simulink model "lab4"  (R2016b)
settings: Solver=VariableStepAuto  StartTime=0.0  StopTime=totaltime  RelTol=1e-3
undefined symbols (not defined in the file or in its folder): h, st
libraries: xbsIndex_r4 x1191
(part 2 of 3)

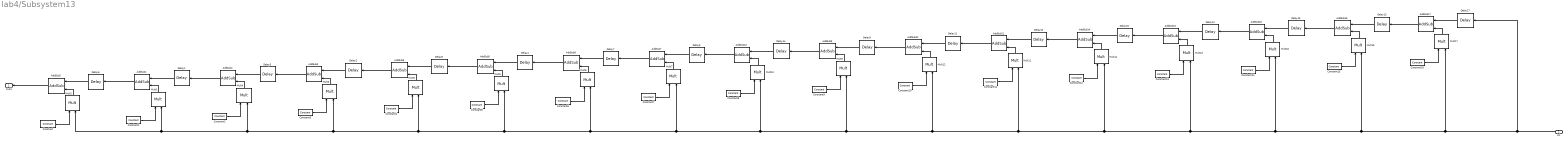
== system lab4/Subsystem13 ==
  In1 : Inport
  AddSub{1..17} (17 alike) : xbsIndex_r4/AddSub  mode=Addition  use_carryin=off  use_carryout=off  en=off  latency=0  precision=User Defined  arith_type="Signed  (2's comp)"  n_bits=17  bin_pt=14  quantization=Truncate  overflow=Wrap  use_behavioral_HDL=off  hw_selection=Fabric  pipelined=off  dbl_ovrd=off  block_type=addsub
  Constant : xbsIndex_r4/Constant  const=h(4,17)  gui_display_data_type=Fixed-point  arith_type=Signed (2's comp)  n_bits=16  bin_pt=14  preci_type=Single  exp_width=8  frac_width=24  explicit_period=off  period=1  equ=P=C  opselect=C  inp2=PCIN>>17  opr=+  inp1=P  carry=CIN  dbl_ovrd=off  block_type=constant
  Constant1 : xbsIndex_r4/Constant  const=h(4,16)  gui_display_data_type=Fixed-point  arith_type=Signed (2's comp)  n_bits=16  bin_pt=14  preci_type=Single  exp_width=8  frac_width=24  explicit_period=off  period=1  equ=P=C  opselect=C  inp2=PCIN>>17  opr=+  inp1=P  carry=CIN  dbl_ovrd=off  block_type=constant
  Constant10 : xbsIndex_r4/Constant  const=h(4,7)  gui_display_data_type=Fixed-point  arith_type=Signed (2's comp)  n_bits=16  bin_pt=14  preci_type=Single  exp_width=8  frac_width=24  explicit_period=off  period=1  equ=P=C  opselect=C  inp2=PCIN>>17  opr=+  inp1=P  carry=CIN  dbl_ovrd=off  block_type=constant
  Constant11 : xbsIndex_r4/Constant  const=h(4,6)  gui_display_data_type=Fixed-point  arith_type=Signed (2's comp)  n_bits=16  bin_pt=14  preci_type=Single  exp_width=8  frac_width=24  explicit_period=off  period=1  equ=P=C  opselect=C  inp2=PCIN>>17  opr=+  inp1=P  carry=CIN  dbl_ovrd=off  block_type=constant
  Constant12 : xbsIndex_r4/Constant  const=h(4,5)  gui_display_data_type=Fixed-point  arith_type=Signed (2's comp)  n_bits=16  bin_pt=14  preci_type=Single  exp_width=8  frac_width=24  explicit_period=off  period=1  equ=P=C  opselect=C  inp2=PCIN>>17  opr=+  inp1=P  carry=CIN  dbl_ovrd=off  block_type=constant
  Constant13 : xbsIndex_r4/Constant  const=h(4,4)  gui_display_data_type=Fixed-point  arith_type=Signed (2's comp)  n_bits=16  bin_pt=14  preci_type=Single  exp_width=8  frac_width=24  explicit_period=off  period=1  equ=P=C  opselect=C  inp2=PCIN>>17  opr=+  inp1=P  carry=CIN  dbl_ovrd=off  block_type=constant
  Constant14 : xbsIndex_r4/Constant  const=h(4,3)  gui_display_data_type=Fixed-point  arith_type=Signed (2's comp)  n_bits=16  bin_pt=14  preci_type=Single  exp_width=8  frac_width=24  explicit_period=off  period=1  equ=P=C  opselect=C  inp2=PCIN>>17  opr=+  inp1=P  carry=CIN  dbl_ovrd=off  block_type=constant
  Constant15 : xbsIndex_r4/Constant  const=h(4,2)  gui_display_data_type=Fixed-point  arith_type=Signed (2's comp)  n_bits=16  bin_pt=14  preci_type=Single  exp_width=8  frac_width=24  explicit_period=off  period=1  equ=P=C  opselect=C  inp2=PCIN>>17  opr=+  inp1=P  carry=CIN  dbl_ovrd=off  block_type=constant
  Constant16 : xbsIndex_r4/Constant  const=h(4,1)  gui_display_data_type=Fixed-point  arith_type=Signed (2's comp)  n_bits=17  bin_pt=14  preci_type=Single  exp_width=8  frac_width=24  explicit_period=off  period=1  equ=P=C  opselect=C  inp2=PCIN>>17  opr=+  inp1=P  carry=CIN  dbl_ovrd=off  block_type=constant
  Constant2 : xbsIndex_r4/Constant  const=h(4,15)  gui_display_data_type=Fixed-point  arith_type=Signed (2's comp)  n_bits=16  bin_pt=14  preci_type=Single  exp_width=8  frac_width=24  explicit_period=off  period=1  equ=P=C  opselect=C  inp2=PCIN>>17  opr=+  inp1=P  carry=CIN  dbl_ovrd=off  block_type=constant
  Constant3 : xbsIndex_r4/Constant  const=h(4,14)  gui_display_data_type=Fixed-point  arith_type=Signed (2's comp)  n_bits=16  bin_pt=14  preci_type=Single  exp_width=8  frac_width=24  explicit_period=off  period=1  equ=P=C  opselect=C  inp2=PCIN>>17  opr=+  inp1=P  carry=CIN  dbl_ovrd=off  block_type=constant
  Constant4 : xbsIndex_r4/Constant  const=h(4,13)  gui_display_data_type=Fixed-point  arith_type=Signed (2's comp)  n_bits=16  bin_pt=14  preci_type=Single  exp_width=8  frac_width=24  explicit_period=off  period=1  equ=P=C  opselect=C  inp2=PCIN>>17  opr=+  inp1=P  carry=CIN  dbl_ovrd=off  block_type=constant
  Constant5 : xbsIndex_r4/Constant  const=h(4,12)  gui_display_data_type=Fixed-point  arith_type=Signed (2's comp)  n_bits=16  bin_pt=14  preci_type=Single  exp_width=8  frac_width=24  explicit_period=off  period=1  equ=P=C  opselect=C  inp2=PCIN>>17  opr=+  inp1=P  carry=CIN  dbl_ovrd=off  block_type=constant
  Constant6 : xbsIndex_r4/Constant  const=h(4,11)  gui_display_data_type=Fixed-point  arith_type=Signed (2's comp)  n_bits=16  bin_pt=14  preci_type=Single  exp_width=8  frac_width=24  explicit_period=off  period=1  equ=P=C  opselect=C  inp2=PCIN>>17  opr=+  inp1=P  carry=CIN  dbl_ovrd=off  block_type=constant
  Constant7 : xbsIndex_r4/Constant  const=h(4,10)  gui_display_data_type=Fixed-point  arith_type=Signed (2's comp)  n_bits=16  bin_pt=14  preci_type=Single  exp_width=8  frac_width=24  explicit_period=off  period=1  equ=P=C  opselect=C  inp2=PCIN>>17  opr=+  inp1=P  carry=CIN  dbl_ovrd=off  block_type=constant
  Constant8 : xbsIndex_r4/Constant  const=h(4,9)  gui_display_data_type=Fixed-point  arith_type=Signed (2's comp)  n_bits=16  bin_pt=14  preci_type=Single  exp_width=8  frac_width=24  explicit_period=off  period=1  equ=P=C  opselect=C  inp2=PCIN>>17  opr=+  inp1=P  carry=CIN  dbl_ovrd=off  block_type=constant
  Constant9 : xbsIndex_r4/Constant  const=h(4,8)  gui_display_data_type=Fixed-point  arith_type=Signed (2's comp)  n_bits=16  bin_pt=14  preci_type=Single  exp_width=8  frac_width=24  explicit_period=off  period=1  equ=P=C  opselect=C  inp2=PCIN>>17  opr=+  inp1=P  carry=CIN  dbl_ovrd=off  block_type=constant
  Delay{1..17} (17 alike) : xbsIndex_r4/Delay  rst=off  infoeditControl=Selection of Reset will increase slice count due to use of real FFs and instead of SRLs  en=off  latency=1  reg_retiming=off  dbl_ovrd=off  block_type=delay
  Mult{1..17} (17 alike) : xbsIndex_r4/Mult  precision=User Defined  arith_type="Signed  (2's comp)"  n_bits=16  bin_pt=14  quantization="Round  (unbiased: +/- Inf)"  overflow=Flag as error  en=off  latency=0  use_behavioral_HDL=off  opt=Speed  use_embedded=on  optimum_pipeline=off  pipeline=on  dbl_ovrd=off  use_rpm=on  placement_style=Triangular  block_type=mult
  Out1 : Outport
  wires:
  Mult2/1 -> AddSub2/2
  AddSub2/1 -> Out1/1
  Delay6/1 -> AddSub2/1
  Constant2/1 -> Mult4/1
  AddSub4/1 -> Delay1/1
  Mult4/1 -> AddSub4/2
  Delay3/1 -> AddSub4/1
  Constant4/1 -> Mult6/1
  AddSub12/1 -> Delay9/1
  Constant3/1 -> Mult3/1
  Mult13/1 -> AddSub13/2
  AddSub13/1 -> Delay16/1
  Delay7/1 -> AddSub8/1
  Constant13/1 -> Mult13/1
  Mult3/1 -> AddSub3/2
  Mult8/1 -> AddSub8/2
  Delay8/1 -> AddSub6/1
  Delay2/1 -> AddSub3/1
  AddSub3/1 -> Delay3/1
  Delay14/1 -> AddSub10/1
  AddSub11/1 -> Delay11/1
  AddSub9/1 -> Delay14/1
  AddSub6/1 -> Delay2/1
  Delay5/1 -> AddSub7/1
  Constant7/1 -> Mult7/1
  Mult5/1 -> AddSub5/2
  Constant5/1 -> Mult5/1
  Mult12/1 -> AddSub12/2
  Mult7/1 -> AddSub7/2
  AddSub7/1 -> Delay7/1
  Delay11/1 -> AddSub12/1
  Mult11/1 -> AddSub11/2
  AddSub8/1 -> Delay4/1
  Delay4/1 -> AddSub5/1
  Constant6/1 -> Mult8/1
  Mult6/1 -> AddSub6/2
  AddSub5/1 -> Delay8/1
  Delay15/1 -> AddSub16/1
  AddSub10/1 -> Delay5/1
  Delay9/1 -> AddSub9/1
  Mult10/1 -> AddSub10/2
  Delay16/1 -> AddSub14/1
  Delay13/1 -> AddSub15/1
  Mult9/1 -> AddSub9/2
  Constant8/1 -> Mult10/1
  Constant15/1 -> Mult15/1
  Constant12/1 -> Mult14/1
  Delay10/1 -> AddSub11/1
  Delay12/1 -> AddSub13/1
  AddSub16/1 -> Delay12/1
  Mult15/1 -> AddSub15/2
  AddSub14/1 -> Delay10/1
  Mult16/1 -> AddSub16/2
  Mult14/1 -> AddSub14/2
  Constant11/1 -> Mult11/1
  Constant9/1 -> Mult9/1
  AddSub15/1 -> Delay15/1
  Constant10/1 -> Mult12/1
  Constant14/1 -> Mult16/1
  In1/1 -> Delay17/1, Mult17/2, Mult15/2, Mult16/2, Mult13/2, Mult14/2, Mult11/2, Mult12/2, Mult9/2, Mult10/2, Mult7/2, Mult8/2, Mult5/2, Mult6/2, Mult3/2, Mult4/2, Mult2/2, Mult1/2
  Delay17/1 -> AddSub17/1
  AddSub17/1 -> Delay13/1
  Mult17/1 -> AddSub17/2
  Constant16/1 -> Mult17/1
  Constant/1 -> Mult2/1
  Delay1/1 -> AddSub1/1
  Mult1/1 -> AddSub1/2
  Constant1/1 -> Mult1/1
  AddSub1/1 -> Delay6/1

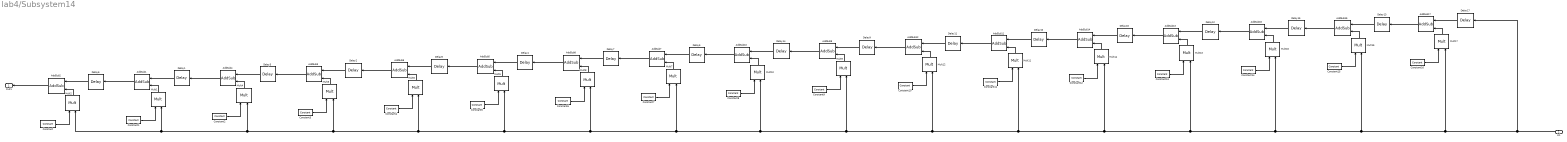
== system lab4/Subsystem14 ==
  In1 : Inport
  AddSub{1..17} (17 alike) : xbsIndex_r4/AddSub  mode=Addition  use_carryin=off  use_carryout=off  en=off  latency=0  precision=User Defined  arith_type="Signed  (2's comp)"  n_bits=17  bin_pt=14  quantization=Truncate  overflow=Wrap  use_behavioral_HDL=off  hw_selection=Fabric  pipelined=off  dbl_ovrd=off  block_type=addsub
  Constant : xbsIndex_r4/Constant  const=h(3,17)  gui_display_data_type=Fixed-point  arith_type=Signed (2's comp)  n_bits=16  bin_pt=14  preci_type=Single  exp_width=8  frac_width=24  explicit_period=off  period=1  equ=P=C  opselect=C  inp2=PCIN>>17  opr=+  inp1=P  carry=CIN  dbl_ovrd=off  block_type=constant
  Constant1 : xbsIndex_r4/Constant  const=h(3,16)  gui_display_data_type=Fixed-point  arith_type=Signed (2's comp)  n_bits=16  bin_pt=14  preci_type=Single  exp_width=8  frac_width=24  explicit_period=off  period=1  equ=P=C  opselect=C  inp2=PCIN>>17  opr=+  inp1=P  carry=CIN  dbl_ovrd=off  block_type=constant
  Constant10 : xbsIndex_r4/Constant  const=h(3,7)  gui_display_data_type=Fixed-point  arith_type=Signed (2's comp)  n_bits=16  bin_pt=14  preci_type=Single  exp_width=8  frac_width=24  explicit_period=off  period=1  equ=P=C  opselect=C  inp2=PCIN>>17  opr=+  inp1=P  carry=CIN  dbl_ovrd=off  block_type=constant
  Constant11 : xbsIndex_r4/Constant  const=h(3,6)  gui_display_data_type=Fixed-point  arith_type=Signed (2's comp)  n_bits=16  bin_pt=14  preci_type=Single  exp_width=8  frac_width=24  explicit_period=off  period=1  equ=P=C  opselect=C  inp2=PCIN>>17  opr=+  inp1=P  carry=CIN  dbl_ovrd=off  block_type=constant
  Constant12 : xbsIndex_r4/Constant  const=h(3,5)  gui_display_data_type=Fixed-point  arith_type=Signed (2's comp)  n_bits=16  bin_pt=14  preci_type=Single  exp_width=8  frac_width=24  explicit_period=off  period=1  equ=P=C  opselect=C  inp2=PCIN>>17  opr=+  inp1=P  carry=CIN  dbl_ovrd=off  block_type=constant
  Constant13 : xbsIndex_r4/Constant  const=h(3,4)  gui_display_data_type=Fixed-point  arith_type=Signed (2's comp)  n_bits=16  bin_pt=14  preci_type=Single  exp_width=8  frac_width=24  explicit_period=off  period=1  equ=P=C  opselect=C  inp2=PCIN>>17  opr=+  inp1=P  carry=CIN  dbl_ovrd=off  block_type=constant
  Constant14 : xbsIndex_r4/Constant  const=h(3,3)  gui_display_data_type=Fixed-point  arith_type=Signed (2's comp)  n_bits=16  bin_pt=14  preci_type=Single  exp_width=8  frac_width=24  explicit_period=off  period=1  equ=P=C  opselect=C  inp2=PCIN>>17  opr=+  inp1=P  carry=CIN  dbl_ovrd=off  block_type=constant
  Constant15 : xbsIndex_r4/Constant  const=h(3,2)  gui_display_data_type=Fixed-point  arith_type=Signed (2's comp)  n_bits=16  bin_pt=14  preci_type=Single  exp_width=8  frac_width=24  explicit_period=off  period=1  equ=P=C  opselect=C  inp2=PCIN>>17  opr=+  inp1=P  carry=CIN  dbl_ovrd=off  block_type=constant
  Constant16 : xbsIndex_r4/Constant  const=h(3,1)  gui_display_data_type=Fixed-point  arith_type=Signed (2's comp)  n_bits=17  bin_pt=14  preci_type=Single  exp_width=8  frac_width=24  explicit_period=off  period=1  equ=P=C  opselect=C  inp2=PCIN>>17  opr=+  inp1=P  carry=CIN  dbl_ovrd=off  block_type=constant
  Constant2 : xbsIndex_r4/Constant  const=h(3,15)  gui_display_data_type=Fixed-point  arith_type=Signed (2's comp)  n_bits=16  bin_pt=14  preci_type=Single  exp_width=8  frac_width=24  explicit_period=off  period=1  equ=P=C  opselect=C  inp2=PCIN>>17  opr=+  inp1=P  carry=CIN  dbl_ovrd=off  block_type=constant
  Constant3 : xbsIndex_r4/Constant  const=h(3,14)  gui_display_data_type=Fixed-point  arith_type=Signed (2's comp)  n_bits=16  bin_pt=14  preci_type=Single  exp_width=8  frac_width=24  explicit_period=off  period=1  equ=P=C  opselect=C  inp2=PCIN>>17  opr=+  inp1=P  carry=CIN  dbl_ovrd=off  block_type=constant
  Constant4 : xbsIndex_r4/Constant  const=h(3,13)  gui_display_data_type=Fixed-point  arith_type=Signed (2's comp)  n_bits=16  bin_pt=14  preci_type=Single  exp_width=8  frac_width=24  explicit_period=off  period=1  equ=P=C  opselect=C  inp2=PCIN>>17  opr=+  inp1=P  carry=CIN  dbl_ovrd=off  block_type=constant
  Constant5 : xbsIndex_r4/Constant  const=h(3,12)  gui_display_data_type=Fixed-point  arith_type=Signed (2's comp)  n_bits=16  bin_pt=14  preci_type=Single  exp_width=8  frac_width=24  explicit_period=off  period=1  equ=P=C  opselect=C  inp2=PCIN>>17  opr=+  inp1=P  carry=CIN  dbl_ovrd=off  block_type=constant
  Constant6 : xbsIndex_r4/Constant  const=h(3,11)  gui_display_data_type=Fixed-point  arith_type=Signed (2's comp)  n_bits=16  bin_pt=14  preci_type=Single  exp_width=8  frac_width=24  explicit_period=off  period=1  equ=P=C  opselect=C  inp2=PCIN>>17  opr=+  inp1=P  carry=CIN  dbl_ovrd=off  block_type=constant
  Constant7 : xbsIndex_r4/Constant  const=h(3,10)  gui_display_data_type=Fixed-point  arith_type=Signed (2's comp)  n_bits=16  bin_pt=14  preci_type=Single  exp_width=8  frac_width=24  explicit_period=off  period=1  equ=P=C  opselect=C  inp2=PCIN>>17  opr=+  inp1=P  carry=CIN  dbl_ovrd=off  block_type=constant
  Constant8 : xbsIndex_r4/Constant  const=h(3,9)  gui_display_data_type=Fixed-point  arith_type=Signed (2's comp)  n_bits=16  bin_pt=14  preci_type=Single  exp_width=8  frac_width=24  explicit_period=off  period=1  equ=P=C  opselect=C  inp2=PCIN>>17  opr=+  inp1=P  carry=CIN  dbl_ovrd=off  block_type=constant
  Constant9 : xbsIndex_r4/Constant  const=h(3,8)  gui_display_data_type=Fixed-point  arith_type=Signed (2's comp)  n_bits=16  bin_pt=14  preci_type=Single  exp_width=8  frac_width=24  explicit_period=off  period=1  equ=P=C  opselect=C  inp2=PCIN>>17  opr=+  inp1=P  carry=CIN  dbl_ovrd=off  block_type=constant
  Delay{1..17} (17 alike) : xbsIndex_r4/Delay  rst=off  infoeditControl=Selection of Reset will increase slice count due to use of real FFs and instead of SRLs  en=off  latency=1  reg_retiming=off  dbl_ovrd=off  block_type=delay
  Mult{1..17} (17 alike) : xbsIndex_r4/Mult  precision=User Defined  arith_type="Signed  (2's comp)"  n_bits=16  bin_pt=14  quantization="Round  (unbiased: +/- Inf)"  overflow=Flag as error  en=off  latency=0  use_behavioral_HDL=off  opt=Speed  use_embedded=on  optimum_pipeline=off  pipeline=on  dbl_ovrd=off  use_rpm=on  placement_style=Triangular  block_type=mult
  Out1 : Outport
  wires:
  Mult2/1 -> AddSub2/2
  AddSub2/1 -> Out1/1
  Delay6/1 -> AddSub2/1
  Constant2/1 -> Mult4/1
  AddSub4/1 -> Delay1/1
  Mult4/1 -> AddSub4/2
  Delay3/1 -> AddSub4/1
  Constant4/1 -> Mult6/1
  AddSub12/1 -> Delay9/1
  Constant3/1 -> Mult3/1
  Mult13/1 -> AddSub13/2
  AddSub13/1 -> Delay16/1
  Delay7/1 -> AddSub8/1
  Constant13/1 -> Mult13/1
  Mult3/1 -> AddSub3/2
  Mult8/1 -> AddSub8/2
  Delay8/1 -> AddSub6/1
  Delay2/1 -> AddSub3/1
  AddSub3/1 -> Delay3/1
  Delay14/1 -> AddSub10/1
  AddSub11/1 -> Delay11/1
  AddSub9/1 -> Delay14/1
  AddSub6/1 -> Delay2/1
  Delay5/1 -> AddSub7/1
  Constant7/1 -> Mult7/1
  Mult5/1 -> AddSub5/2
  Constant5/1 -> Mult5/1
  Mult12/1 -> AddSub12/2
  Mult7/1 -> AddSub7/2
  AddSub7/1 -> Delay7/1
  Delay11/1 -> AddSub12/1
  Mult11/1 -> AddSub11/2
  AddSub8/1 -> Delay4/1
  Delay4/1 -> AddSub5/1
  Constant6/1 -> Mult8/1
  Mult6/1 -> AddSub6/2
  AddSub5/1 -> Delay8/1
  Delay15/1 -> AddSub16/1
  AddSub10/1 -> Delay5/1
  Delay9/1 -> AddSub9/1
  Mult10/1 -> AddSub10/2
  Delay16/1 -> AddSub14/1
  Delay13/1 -> AddSub15/1
  Mult9/1 -> AddSub9/2
  Constant8/1 -> Mult10/1
  Constant15/1 -> Mult15/1
  Constant12/1 -> Mult14/1
  Delay10/1 -> AddSub11/1
  Delay12/1 -> AddSub13/1
  AddSub16/1 -> Delay12/1
  Mult15/1 -> AddSub15/2
  AddSub14/1 -> Delay10/1
  Mult16/1 -> AddSub16/2
  Mult14/1 -> AddSub14/2
  Constant11/1 -> Mult11/1
  Constant9/1 -> Mult9/1
  AddSub15/1 -> Delay15/1
  Constant10/1 -> Mult12/1
  Constant14/1 -> Mult16/1
  In1/1 -> Delay17/1, Mult17/2, Mult15/2, Mult16/2, Mult13/2, Mult14/2, Mult11/2, Mult12/2, Mult9/2, Mult10/2, Mult7/2, Mult8/2, Mult5/2, Mult6/2, Mult3/2, Mult4/2, Mult2/2, Mult1/2
  Delay17/1 -> AddSub17/1
  AddSub17/1 -> Delay13/1
  Mult17/1 -> AddSub17/2
  Constant16/1 -> Mult17/1
  Constant/1 -> Mult2/1
  Delay1/1 -> AddSub1/1
  Mult1/1 -> AddSub1/2
  Constant1/1 -> Mult1/1
  AddSub1/1 -> Delay6/1

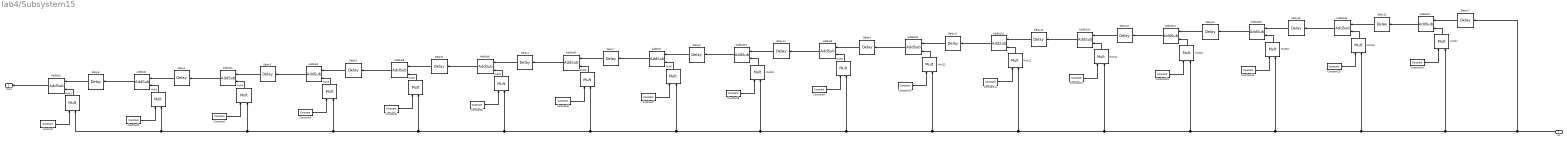
== system lab4/Subsystem15 ==
  In1 : Inport
  AddSub{1..17} (17 alike) : xbsIndex_r4/AddSub  mode=Addition  use_carryin=off  use_carryout=off  en=off  latency=0  precision=User Defined  arith_type="Signed  (2's comp)"  n_bits=17  bin_pt=14  quantization=Truncate  overflow=Wrap  use_behavioral_HDL=off  hw_selection=Fabric  pipelined=off  dbl_ovrd=off  block_type=addsub
  Constant : xbsIndex_r4/Constant  const=h(2,17)  gui_display_data_type=Fixed-point  arith_type=Signed (2's comp)  n_bits=16  bin_pt=14  preci_type=Single  exp_width=8  frac_width=24  explicit_period=off  period=1  equ=P=C  opselect=C  inp2=PCIN>>17  opr=+  inp1=P  carry=CIN  dbl_ovrd=off  block_type=constant
  Constant1 : xbsIndex_r4/Constant  const=h(2,16)  gui_display_data_type=Fixed-point  arith_type=Signed (2's comp)  n_bits=16  bin_pt=14  preci_type=Single  exp_width=8  frac_width=24  explicit_period=off  period=1  equ=P=C  opselect=C  inp2=PCIN>>17  opr=+  inp1=P  carry=CIN  dbl_ovrd=off  block_type=constant
  Constant10 : xbsIndex_r4/Constant  const=h(2,7)  gui_display_data_type=Fixed-point  arith_type=Signed (2's comp)  n_bits=16  bin_pt=14  preci_type=Single  exp_width=8  frac_width=24  explicit_period=off  period=1  equ=P=C  opselect=C  inp2=PCIN>>17  opr=+  inp1=P  carry=CIN  dbl_ovrd=off  block_type=constant
  Constant11 : xbsIndex_r4/Constant  const=h(2,6)  gui_display_data_type=Fixed-point  arith_type=Signed (2's comp)  n_bits=16  bin_pt=14  preci_type=Single  exp_width=8  frac_width=24  explicit_period=off  period=1  equ=P=C  opselect=C  inp2=PCIN>>17  opr=+  inp1=P  carry=CIN  dbl_ovrd=off  block_type=constant
  Constant12 : xbsIndex_r4/Constant  const=h(2,5)  gui_display_data_type=Fixed-point  arith_type=Signed (2's comp)  n_bits=16  bin_pt=14  preci_type=Single  exp_width=8  frac_width=24  explicit_period=off  period=1  equ=P=C  opselect=C  inp2=PCIN>>17  opr=+  inp1=P  carry=CIN  dbl_ovrd=off  block_type=constant
  Constant13 : xbsIndex_r4/Constant  const=h(2,4)  gui_display_data_type=Fixed-point  arith_type=Signed (2's comp)  n_bits=16  bin_pt=14  preci_type=Single  exp_width=8  frac_width=24  explicit_period=off  period=1  equ=P=C  opselect=C  inp2=PCIN>>17  opr=+  inp1=P  carry=CIN  dbl_ovrd=off  block_type=constant
  Constant14 : xbsIndex_r4/Constant  const=h(2,3)  gui_display_data_type=Fixed-point  arith_type=Signed (2's comp)  n_bits=16  bin_pt=14  preci_type=Single  exp_width=8  frac_width=24  explicit_period=off  period=1  equ=P=C  opselect=C  inp2=PCIN>>17  opr=+  inp1=P  carry=CIN  dbl_ovrd=off  block_type=constant
  Constant15 : xbsIndex_r4/Constant  const=h(2,2)  gui_display_data_type=Fixed-point  arith_type=Signed (2's comp)  n_bits=16  bin_pt=14  preci_type=Single  exp_width=8  frac_width=24  explicit_period=off  period=1  equ=P=C  opselect=C  inp2=PCIN>>17  opr=+  inp1=P  carry=CIN  dbl_ovrd=off  block_type=constant
  Constant16 : xbsIndex_r4/Constant  const=h(2,1)  gui_display_data_type=Fixed-point  arith_type=Signed (2's comp)  n_bits=17  bin_pt=14  preci_type=Single  exp_width=8  frac_width=24  explicit_period=off  period=1  equ=P=C  opselect=C  inp2=PCIN>>17  opr=+  inp1=P  carry=CIN  dbl_ovrd=off  block_type=constant
  Constant2 : xbsIndex_r4/Constant  const=h(2,15)  gui_display_data_type=Fixed-point  arith_type=Signed (2's comp)  n_bits=16  bin_pt=14  preci_type=Single  exp_width=8  frac_width=24  explicit_period=off  period=1  equ=P=C  opselect=C  inp2=PCIN>>17  opr=+  inp1=P  carry=CIN  dbl_ovrd=off  block_type=constant
  Constant3 : xbsIndex_r4/Constant  const=h(2,14)  gui_display_data_type=Fixed-point  arith_type=Signed (2's comp)  n_bits=16  bin_pt=14  preci_type=Single  exp_width=8  frac_width=24  explicit_period=off  period=1  equ=P=C  opselect=C  inp2=PCIN>>17  opr=+  inp1=P  carry=CIN  dbl_ovrd=off  block_type=constant
  Constant4 : xbsIndex_r4/Constant  const=h(2,13)  gui_display_data_type=Fixed-point  arith_type=Signed (2's comp)  n_bits=16  bin_pt=14  preci_type=Single  exp_width=8  frac_width=24  explicit_period=off  period=1  equ=P=C  opselect=C  inp2=PCIN>>17  opr=+  inp1=P  carry=CIN  dbl_ovrd=off  block_type=constant
  Constant5 : xbsIndex_r4/Constant  const=h(2,12)  gui_display_data_type=Fixed-point  arith_type=Signed (2's comp)  n_bits=16  bin_pt=14  preci_type=Single  exp_width=8  frac_width=24  explicit_period=off  period=1  equ=P=C  opselect=C  inp2=PCIN>>17  opr=+  inp1=P  carry=CIN  dbl_ovrd=off  block_type=constant
  Constant6 : xbsIndex_r4/Constant  const=h(2,11)  gui_display_data_type=Fixed-point  arith_type=Signed (2's comp)  n_bits=16  bin_pt=14  preci_type=Single  exp_width=8  frac_width=24  explicit_period=off  period=1  equ=P=C  opselect=C  inp2=PCIN>>17  opr=+  inp1=P  carry=CIN  dbl_ovrd=off  block_type=constant
  Constant7 : xbsIndex_r4/Constant  const=h(2,10)  gui_display_data_type=Fixed-point  arith_type=Signed (2's comp)  n_bits=16  bin_pt=14  preci_type=Single  exp_width=8  frac_width=24  explicit_period=off  period=1  equ=P=C  opselect=C  inp2=PCIN>>17  opr=+  inp1=P  carry=CIN  dbl_ovrd=off  block_type=constant
  Constant8 : xbsIndex_r4/Constant  const=h(2,9)  gui_display_data_type=Fixed-point  arith_type=Signed (2's comp)  n_bits=16  bin_pt=14  preci_type=Single  exp_width=8  frac_width=24  explicit_period=off  period=1  equ=P=C  opselect=C  inp2=PCIN>>17  opr=+  inp1=P  carry=CIN  dbl_ovrd=off  block_type=constant
  Constant9 : xbsIndex_r4/Constant  const=h(2,8)  gui_display_data_type=Fixed-point  arith_type=Signed (2's comp)  n_bits=16  bin_pt=14  preci_type=Single  exp_width=8  frac_width=24  explicit_period=off  period=1  equ=P=C  opselect=C  inp2=PCIN>>17  opr=+  inp1=P  carry=CIN  dbl_ovrd=off  block_type=constant
  Delay{1..17} (17 alike) : xbsIndex_r4/Delay  rst=off  infoeditControl=Selection of Reset will increase slice count due to use of real FFs and instead of SRLs  en=off  latency=1  reg_retiming=off  dbl_ovrd=off  block_type=delay
  Mult{1..17} (17 alike) : xbsIndex_r4/Mult  precision=User Defined  arith_type="Signed  (2's comp)"  n_bits=16  bin_pt=14  quantization="Round  (unbiased: +/- Inf)"  overflow=Flag as error  en=off  latency=0  use_behavioral_HDL=off  opt=Speed  use_embedded=on  optimum_pipeline=off  pipeline=on  dbl_ovrd=off  use_rpm=on  placement_style=Triangular  block_type=mult
  Out1 : Outport
  wires:
  Mult2/1 -> AddSub2/2
  AddSub2/1 -> Out1/1
  Delay6/1 -> AddSub2/1
  Constant2/1 -> Mult4/1
  AddSub4/1 -> Delay1/1
  Mult4/1 -> AddSub4/2
  Delay3/1 -> AddSub4/1
  Constant4/1 -> Mult6/1
  AddSub12/1 -> Delay9/1
  Constant3/1 -> Mult3/1
  Mult13/1 -> AddSub13/2
  AddSub13/1 -> Delay16/1
  Delay7/1 -> AddSub8/1
  Constant13/1 -> Mult13/1
  Mult3/1 -> AddSub3/2
  Mult8/1 -> AddSub8/2
  Delay8/1 -> AddSub6/1
  Delay2/1 -> AddSub3/1
  AddSub3/1 -> Delay3/1
  Delay14/1 -> AddSub10/1
  AddSub11/1 -> Delay11/1
  AddSub9/1 -> Delay14/1
  AddSub6/1 -> Delay2/1
  Delay5/1 -> AddSub7/1
  Constant7/1 -> Mult7/1
  Mult5/1 -> AddSub5/2
  Constant5/1 -> Mult5/1
  Mult12/1 -> AddSub12/2
  Mult7/1 -> AddSub7/2
  AddSub7/1 -> Delay7/1
  Delay11/1 -> AddSub12/1
  Mult11/1 -> AddSub11/2
  AddSub8/1 -> Delay4/1
  Delay4/1 -> AddSub5/1
  Constant6/1 -> Mult8/1
  Mult6/1 -> AddSub6/2
  AddSub5/1 -> Delay8/1
  Delay15/1 -> AddSub16/1
  AddSub10/1 -> Delay5/1
  Delay9/1 -> AddSub9/1
  Mult10/1 -> AddSub10/2
  Delay16/1 -> AddSub14/1
  Delay13/1 -> AddSub15/1
  Mult9/1 -> AddSub9/2
  Constant8/1 -> Mult10/1
  Constant15/1 -> Mult15/1
  Constant12/1 -> Mult14/1
  Delay10/1 -> AddSub11/1
  Delay12/1 -> AddSub13/1
  AddSub16/1 -> Delay12/1
  Mult15/1 -> AddSub15/2
  AddSub14/1 -> Delay10/1
  Mult16/1 -> AddSub16/2
  Mult14/1 -> AddSub14/2
  Constant11/1 -> Mult11/1
  Constant9/1 -> Mult9/1
  AddSub15/1 -> Delay15/1
  Constant10/1 -> Mult12/1
  Constant14/1 -> Mult16/1
  In1/1 -> Delay17/1, Mult17/2, Mult15/2, Mult16/2, Mult13/2, Mult14/2, Mult11/2, Mult12/2, Mult9/2, Mult10/2, Mult7/2, Mult8/2, Mult5/2, Mult6/2, Mult3/2, Mult4/2, Mult2/2, Mult1/2
  Delay17/1 -> AddSub17/1
  AddSub17/1 -> Delay13/1
  Mult17/1 -> AddSub17/2
  Constant16/1 -> Mult17/1
  Constant/1 -> Mult2/1
  Delay1/1 -> AddSub1/1
  Mult1/1 -> AddSub1/2
  Constant1/1 -> Mult1/1
  AddSub1/1 -> Delay6/1

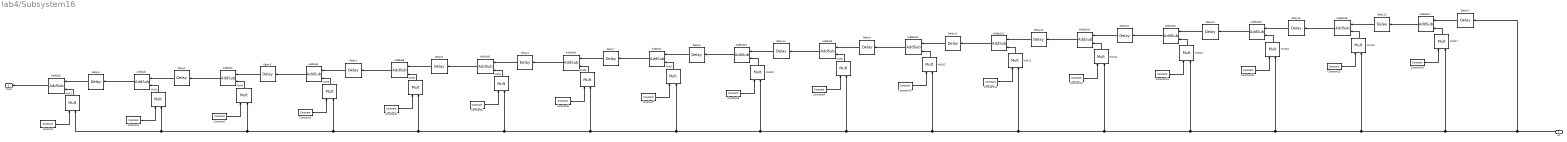
== system lab4/Subsystem16 ==
  In1 : Inport
  AddSub{1..17} (17 alike) : xbsIndex_r4/AddSub  mode=Addition  use_carryin=off  use_carryout=off  en=off  latency=0  precision=User Defined  arith_type="Signed  (2's comp)"  n_bits=17  bin_pt=14  quantization=Truncate  overflow=Wrap  use_behavioral_HDL=off  hw_selection=Fabric  pipelined=off  dbl_ovrd=off  block_type=addsub
  Constant : xbsIndex_r4/Constant  const=h(1,17)  gui_display_data_type=Fixed-point  arith_type=Signed (2's comp)  n_bits=16  bin_pt=14  preci_type=Single  exp_width=8  frac_width=24  explicit_period=off  period=1  equ=P=C  opselect=C  inp2=PCIN>>17  opr=+  inp1=P  carry=CIN  dbl_ovrd=off  block_type=constant
  Constant1 : xbsIndex_r4/Constant  const=h(1,16)  gui_display_data_type=Fixed-point  arith_type=Signed (2's comp)  n_bits=16  bin_pt=14  preci_type=Single  exp_width=8  frac_width=24  explicit_period=off  period=1  equ=P=C  opselect=C  inp2=PCIN>>17  opr=+  inp1=P  carry=CIN  dbl_ovrd=off  block_type=constant
  Constant10 : xbsIndex_r4/Constant  const=h(1,7)  gui_display_data_type=Fixed-point  arith_type=Signed (2's comp)  n_bits=16  bin_pt=14  preci_type=Single  exp_width=8  frac_width=24  explicit_period=off  period=1  equ=P=C  opselect=C  inp2=PCIN>>17  opr=+  inp1=P  carry=CIN  dbl_ovrd=off  block_type=constant
  Constant11 : xbsIndex_r4/Constant  const=h(1,6)  gui_display_data_type=Fixed-point  arith_type=Signed (2's comp)  n_bits=16  bin_pt=14  preci_type=Single  exp_width=8  frac_width=24  explicit_period=off  period=1  equ=P=C  opselect=C  inp2=PCIN>>17  opr=+  inp1=P  carry=CIN  dbl_ovrd=off  block_type=constant
  Constant12 : xbsIndex_r4/Constant  const=h(1,5)  gui_display_data_type=Fixed-point  arith_type=Signed (2's comp)  n_bits=16  bin_pt=14  preci_type=Single  exp_width=8  frac_width=24  explicit_period=off  period=1  equ=P=C  opselect=C  inp2=PCIN>>17  opr=+  inp1=P  carry=CIN  dbl_ovrd=off  block_type=constant
  Constant13 : xbsIndex_r4/Constant  const=h(1,4)  gui_display_data_type=Fixed-point  arith_type=Signed (2's comp)  n_bits=16  bin_pt=14  preci_type=Single  exp_width=8  frac_width=24  explicit_period=off  period=1  equ=P=C  opselect=C  inp2=PCIN>>17  opr=+  inp1=P  carry=CIN  dbl_ovrd=off  block_type=constant
  Constant14 : xbsIndex_r4/Constant  const=h(1,3)  gui_display_data_type=Fixed-point  arith_type=Signed (2's comp)  n_bits=16  bin_pt=14  preci_type=Single  exp_width=8  frac_width=24  explicit_period=off  period=1  equ=P=C  opselect=C  inp2=PCIN>>17  opr=+  inp1=P  carry=CIN  dbl_ovrd=off  block_type=constant
  Constant15 : xbsIndex_r4/Constant  const=h(1,2)  gui_display_data_type=Fixed-point  arith_type=Signed (2's comp)  n_bits=16  bin_pt=14  preci_type=Single  exp_width=8  frac_width=24  explicit_period=off  period=1  equ=P=C  opselect=C  inp2=PCIN>>17  opr=+  inp1=P  carry=CIN  dbl_ovrd=off  block_type=constant
  Constant16 : xbsIndex_r4/Constant  const=h(1,1)  gui_display_data_type=Fixed-point  arith_type=Signed (2's comp)  n_bits=17  bin_pt=14  preci_type=Single  exp_width=8  frac_width=24  explicit_period=off  period=1  equ=P=C  opselect=C  inp2=PCIN>>17  opr=+  inp1=P  carry=CIN  dbl_ovrd=off  block_type=constant
  Constant2 : xbsIndex_r4/Constant  const=h(1,15)  gui_display_data_type=Fixed-point  arith_type=Signed (2's comp)  n_bits=16  bin_pt=14  preci_type=Single  exp_width=8  frac_width=24  explicit_period=off  period=1  equ=P=C  opselect=C  inp2=PCIN>>17  opr=+  inp1=P  carry=CIN  dbl_ovrd=off  block_type=constant
  Constant3 : xbsIndex_r4/Constant  const=h(1,14)  gui_display_data_type=Fixed-point  arith_type=Signed (2's comp)  n_bits=16  bin_pt=14  preci_type=Single  exp_width=8  frac_width=24  explicit_period=off  period=1  equ=P=C  opselect=C  inp2=PCIN>>17  opr=+  inp1=P  carry=CIN  dbl_ovrd=off  block_type=constant
  Constant4 : xbsIndex_r4/Constant  const=h(1,13)  gui_display_data_type=Fixed-point  arith_type=Signed (2's comp)  n_bits=16  bin_pt=14  preci_type=Single  exp_width=8  frac_width=24  explicit_period=off  period=1  equ=P=C  opselect=C  inp2=PCIN>>17  opr=+  inp1=P  carry=CIN  dbl_ovrd=off  block_type=constant
  Constant5 : xbsIndex_r4/Constant  const=h(1,12)  gui_display_data_type=Fixed-point  arith_type=Signed (2's comp)  n_bits=16  bin_pt=14  preci_type=Single  exp_width=8  frac_width=24  explicit_period=off  period=1  equ=P=C  opselect=C  inp2=PCIN>>17  opr=+  inp1=P  carry=CIN  dbl_ovrd=off  block_type=constant
  Constant6 : xbsIndex_r4/Constant  const=h(1,11)  gui_display_data_type=Fixed-point  arith_type=Signed (2's comp)  n_bits=16  bin_pt=14  preci_type=Single  exp_width=8  frac_width=24  explicit_period=off  period=1  equ=P=C  opselect=C  inp2=PCIN>>17  opr=+  inp1=P  carry=CIN  dbl_ovrd=off  block_type=constant
  Constant7 : xbsIndex_r4/Constant  const=h(1,10)  gui_display_data_type=Fixed-point  arith_type=Signed (2's comp)  n_bits=16  bin_pt=14  preci_type=Single  exp_width=8  frac_width=24  explicit_period=off  period=1  equ=P=C  opselect=C  inp2=PCIN>>17  opr=+  inp1=P  carry=CIN  dbl_ovrd=off  block_type=constant
  Constant8 : xbsIndex_r4/Constant  const=h(1,9)  gui_display_data_type=Fixed-point  arith_type=Signed (2's comp)  n_bits=16  bin_pt=14  preci_type=Single  exp_width=8  frac_width=24  explicit_period=off  period=1  equ=P=C  opselect=C  inp2=PCIN>>17  opr=+  inp1=P  carry=CIN  dbl_ovrd=off  block_type=constant
  Constant9 : xbsIndex_r4/Constant  const=h(1,8)  gui_display_data_type=Fixed-point  arith_type=Signed (2's comp)  n_bits=16  bin_pt=14  preci_type=Single  exp_width=8  frac_width=24  explicit_period=off  period=1  equ=P=C  opselect=C  inp2=PCIN>>17  opr=+  inp1=P  carry=CIN  dbl_ovrd=off  block_type=constant
  Delay{1..17} (17 alike) : xbsIndex_r4/Delay  rst=off  infoeditControl=Selection of Reset will increase slice count due to use of real FFs and instead of SRLs  en=off  latency=1  reg_retiming=off  dbl_ovrd=off  block_type=delay
  Mult{1..17} (17 alike) : xbsIndex_r4/Mult  precision=User Defined  arith_type="Signed  (2's comp)"  n_bits=16  bin_pt=14  quantization="Round  (unbiased: +/- Inf)"  overflow=Flag as error  en=off  latency=0  use_behavioral_HDL=off  opt=Speed  use_embedded=on  optimum_pipeline=off  pipeline=on  dbl_ovrd=off  use_rpm=on  placement_style=Triangular  block_type=mult
  Out1 : Outport
  wires:
  Mult2/1 -> AddSub2/2
  AddSub2/1 -> Out1/1
  Delay6/1 -> AddSub2/1
  Constant2/1 -> Mult4/1
  AddSub4/1 -> Delay1/1
  Mult4/1 -> AddSub4/2
  Delay3/1 -> AddSub4/1
  Constant4/1 -> Mult6/1
  AddSub12/1 -> Delay9/1
  Constant3/1 -> Mult3/1
  Mult13/1 -> AddSub13/2
  AddSub13/1 -> Delay16/1
  Delay7/1 -> AddSub8/1
  Constant13/1 -> Mult13/1
  Mult3/1 -> AddSub3/2
  Mult8/1 -> AddSub8/2
  Delay8/1 -> AddSub6/1
  Delay2/1 -> AddSub3/1
  AddSub3/1 -> Delay3/1
  Delay14/1 -> AddSub10/1
  AddSub11/1 -> Delay11/1
  AddSub9/1 -> Delay14/1
  AddSub6/1 -> Delay2/1
  Delay5/1 -> AddSub7/1
  Constant7/1 -> Mult7/1
  Mult5/1 -> AddSub5/2
  Constant5/1 -> Mult5/1
  Mult12/1 -> AddSub12/2
  Mult7/1 -> AddSub7/2
  AddSub7/1 -> Delay7/1
  Delay11/1 -> AddSub12/1
  Mult11/1 -> AddSub11/2
  AddSub8/1 -> Delay4/1
  Delay4/1 -> AddSub5/1
  Constant6/1 -> Mult8/1
  Mult6/1 -> AddSub6/2
  AddSub5/1 -> Delay8/1
  Delay15/1 -> AddSub16/1
  AddSub10/1 -> Delay5/1
  Delay9/1 -> AddSub9/1
  Mult10/1 -> AddSub10/2
  Delay16/1 -> AddSub14/1
  Delay13/1 -> AddSub15/1
  Mult9/1 -> AddSub9/2
  Constant8/1 -> Mult10/1
  Constant15/1 -> Mult15/1
  Constant12/1 -> Mult14/1
  Delay10/1 -> AddSub11/1
  Delay12/1 -> AddSub13/1
  AddSub16/1 -> Delay12/1
  Mult15/1 -> AddSub15/2
  AddSub14/1 -> Delay10/1
  Mult16/1 -> AddSub16/2
  Mult14/1 -> AddSub14/2
  Constant11/1 -> Mult11/1
  Constant9/1 -> Mult9/1
  AddSub15/1 -> Delay15/1
  Constant10/1 -> Mult12/1
  Constant14/1 -> Mult16/1
  In1/1 -> Delay17/1, Mult17/2, Mult15/2, Mult16/2, Mult13/2, Mult14/2, Mult11/2, Mult12/2, Mult9/2, Mult10/2, Mult7/2, Mult8/2, Mult5/2, Mult6/2, Mult3/2, Mult4/2, Mult2/2, Mult1/2
  Delay17/1 -> AddSub17/1
  AddSub17/1 -> Delay13/1
  Mult17/1 -> AddSub17/2
  Constant16/1 -> Mult17/1
  Constant/1 -> Mult2/1
  Delay1/1 -> AddSub1/1
  Mult1/1 -> AddSub1/2
  Constant1/1 -> Mult1/1
  AddSub1/1 -> Delay6/1

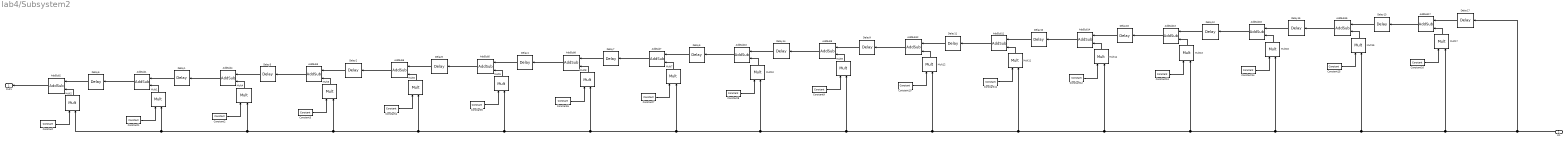
== system lab4/Subsystem2 ==
  In1 : Inport
  AddSub{1..17} (17 alike) : xbsIndex_r4/AddSub  mode=Addition  use_carryin=off  use_carryout=off  en=off  latency=0  precision=User Defined  arith_type="Signed  (2's comp)"  n_bits=17  bin_pt=14  quantization=Truncate  overflow=Wrap  use_behavioral_HDL=off  hw_selection=Fabric  pipelined=off  dbl_ovrd=off  block_type=addsub
  Constant : xbsIndex_r4/Constant  const=h(15,17)  gui_display_data_type=Fixed-point  arith_type=Signed (2's comp)  n_bits=16  bin_pt=14  preci_type=Single  exp_width=8  frac_width=24  explicit_period=off  period=1  equ=P=C  opselect=C  inp2=PCIN>>17  opr=+  inp1=P  carry=CIN  dbl_ovrd=off  block_type=constant
  Constant1 : xbsIndex_r4/Constant  const=h(15,16)  gui_display_data_type=Fixed-point  arith_type=Signed (2's comp)  n_bits=16  bin_pt=14  preci_type=Single  exp_width=8  frac_width=24  explicit_period=off  period=1  equ=P=C  opselect=C  inp2=PCIN>>17  opr=+  inp1=P  carry=CIN  dbl_ovrd=off  block_type=constant
  Constant10 : xbsIndex_r4/Constant  const=h(15,7)  gui_display_data_type=Fixed-point  arith_type=Signed (2's comp)  n_bits=16  bin_pt=14  preci_type=Single  exp_width=8  frac_width=24  explicit_period=off  period=1  equ=P=C  opselect=C  inp2=PCIN>>17  opr=+  inp1=P  carry=CIN  dbl_ovrd=off  block_type=constant
  Constant11 : xbsIndex_r4/Constant  const=h(15,6)  gui_display_data_type=Fixed-point  arith_type=Signed (2's comp)  n_bits=16  bin_pt=14  preci_type=Single  exp_width=8  frac_width=24  explicit_period=off  period=1  equ=P=C  opselect=C  inp2=PCIN>>17  opr=+  inp1=P  carry=CIN  dbl_ovrd=off  block_type=constant
  Constant12 : xbsIndex_r4/Constant  const=h(15,5)  gui_display_data_type=Fixed-point  arith_type=Signed (2's comp)  n_bits=16  bin_pt=14  preci_type=Single  exp_width=8  frac_width=24  explicit_period=off  period=1  equ=P=C  opselect=C  inp2=PCIN>>17  opr=+  inp1=P  carry=CIN  dbl_ovrd=off  block_type=constant
  Constant13 : xbsIndex_r4/Constant  const=h(15,4)  gui_display_data_type=Fixed-point  arith_type=Signed (2's comp)  n_bits=16  bin_pt=14  preci_type=Single  exp_width=8  frac_width=24  explicit_period=off  period=1  equ=P=C  opselect=C  inp2=PCIN>>17  opr=+  inp1=P  carry=CIN  dbl_ovrd=off  block_type=constant
  Constant14 : xbsIndex_r4/Constant  const=h(15,3)  gui_display_data_type=Fixed-point  arith_type=Signed (2's comp)  n_bits=16  bin_pt=14  preci_type=Single  exp_width=8  frac_width=24  explicit_period=off  period=1  equ=P=C  opselect=C  inp2=PCIN>>17  opr=+  inp1=P  carry=CIN  dbl_ovrd=off  block_type=constant
  Constant15 : xbsIndex_r4/Constant  const=h(15,2)  gui_display_data_type=Fixed-point  arith_type=Signed (2's comp)  n_bits=16  bin_pt=14  preci_type=Single  exp_width=8  frac_width=24  explicit_period=off  period=1  equ=P=C  opselect=C  inp2=PCIN>>17  opr=+  inp1=P  carry=CIN  dbl_ovrd=off  block_type=constant
  Constant16 : xbsIndex_r4/Constant  const=h(15,1)  gui_display_data_type=Fixed-point  arith_type=Signed (2's comp)  n_bits=17  bin_pt=14  preci_type=Single  exp_width=8  frac_width=24  explicit_period=off  period=1  equ=P=C  opselect=C  inp2=PCIN>>17  opr=+  inp1=P  carry=CIN  dbl_ovrd=off  block_type=constant
  Constant2 : xbsIndex_r4/Constant  const=h(15,15)  gui_display_data_type=Fixed-point  arith_type=Signed (2's comp)  n_bits=16  bin_pt=14  preci_type=Single  exp_width=8  frac_width=24  explicit_period=off  period=1  equ=P=C  opselect=C  inp2=PCIN>>17  opr=+  inp1=P  carry=CIN  dbl_ovrd=off  block_type=constant
  Constant3 : xbsIndex_r4/Constant  const=h(15,14)  gui_display_data_type=Fixed-point  arith_type=Signed (2's comp)  n_bits=16  bin_pt=14  preci_type=Single  exp_width=8  frac_width=24  explicit_period=off  period=1  equ=P=C  opselect=C  inp2=PCIN>>17  opr=+  inp1=P  carry=CIN  dbl_ovrd=off  block_type=constant
  Constant4 : xbsIndex_r4/Constant  const=h(15,13)  gui_display_data_type=Fixed-point  arith_type=Signed (2's comp)  n_bits=16  bin_pt=14  preci_type=Single  exp_width=8  frac_width=24  explicit_period=off  period=1  equ=P=C  opselect=C  inp2=PCIN>>17  opr=+  inp1=P  carry=CIN  dbl_ovrd=off  block_type=constant
  Constant5 : xbsIndex_r4/Constant  const=h(15,12)  gui_display_data_type=Fixed-point  arith_type=Signed (2's comp)  n_bits=16  bin_pt=14  preci_type=Single  exp_width=8  frac_width=24  explicit_period=off  period=1  equ=P=C  opselect=C  inp2=PCIN>>17  opr=+  inp1=P  carry=CIN  dbl_ovrd=off  block_type=constant
  Constant6 : xbsIndex_r4/Constant  const=h(15,11)  gui_display_data_type=Fixed-point  arith_type=Signed (2's comp)  n_bits=16  bin_pt=14  preci_type=Single  exp_width=8  frac_width=24  explicit_period=off  period=1  equ=P=C  opselect=C  inp2=PCIN>>17  opr=+  inp1=P  carry=CIN  dbl_ovrd=off  block_type=constant
  Constant7 : xbsIndex_r4/Constant  const=h(15,10)  gui_display_data_type=Fixed-point  arith_type=Signed (2's comp)  n_bits=16  bin_pt=14  preci_type=Single  exp_width=8  frac_width=24  explicit_period=off  period=1  equ=P=C  opselect=C  inp2=PCIN>>17  opr=+  inp1=P  carry=CIN  dbl_ovrd=off  block_type=constant
  Constant8 : xbsIndex_r4/Constant  const=h(15,9)  gui_display_data_type=Fixed-point  arith_type=Signed (2's comp)  n_bits=16  bin_pt=14  preci_type=Single  exp_width=8  frac_width=24  explicit_period=off  period=1  equ=P=C  opselect=C  inp2=PCIN>>17  opr=+  inp1=P  carry=CIN  dbl_ovrd=off  block_type=constant
  Constant9 : xbsIndex_r4/Constant  const=h(15,8)  gui_display_data_type=Fixed-point  arith_type=Signed (2's comp)  n_bits=16  bin_pt=14  preci_type=Single  exp_width=8  frac_width=24  explicit_period=off  period=1  equ=P=C  opselect=C  inp2=PCIN>>17  opr=+  inp1=P  carry=CIN  dbl_ovrd=off  block_type=constant
  Delay{1..17} (17 alike) : xbsIndex_r4/Delay  rst=off  infoeditControl=Selection of Reset will increase slice count due to use of real FFs and instead of SRLs  en=off  latency=1  reg_retiming=off  dbl_ovrd=off  block_type=delay
  Mult{1..17} (17 alike) : xbsIndex_r4/Mult  precision=User Defined  arith_type="Signed  (2's comp)"  n_bits=16  bin_pt=14  quantization="Round  (unbiased: +/- Inf)"  overflow=Flag as error  en=off  latency=0  use_behavioral_HDL=off  opt=Speed  use_embedded=on  optimum_pipeline=off  pipeline=on  dbl_ovrd=off  use_rpm=on  placement_style=Triangular  block_type=mult
  Out1 : Outport
  wires:
  Mult2/1 -> AddSub2/2
  AddSub2/1 -> Out1/1
  Delay6/1 -> AddSub2/1
  Constant2/1 -> Mult4/1
  AddSub4/1 -> Delay1/1
  Mult4/1 -> AddSub4/2
  Delay3/1 -> AddSub4/1
  Constant4/1 -> Mult6/1
  AddSub12/1 -> Delay9/1
  Constant3/1 -> Mult3/1
  Mult13/1 -> AddSub13/2
  AddSub13/1 -> Delay16/1
  Delay7/1 -> AddSub8/1
  Constant13/1 -> Mult13/1
  Mult3/1 -> AddSub3/2
  Mult8/1 -> AddSub8/2
  Delay8/1 -> AddSub6/1
  Delay2/1 -> AddSub3/1
  AddSub3/1 -> Delay3/1
  Delay14/1 -> AddSub10/1
  AddSub11/1 -> Delay11/1
  AddSub9/1 -> Delay14/1
  AddSub6/1 -> Delay2/1
  Delay5/1 -> AddSub7/1
  Constant7/1 -> Mult7/1
  Mult5/1 -> AddSub5/2
  Constant5/1 -> Mult5/1
  Mult12/1 -> AddSub12/2
  Mult7/1 -> AddSub7/2
  AddSub7/1 -> Delay7/1
  Delay11/1 -> AddSub12/1
  Mult11/1 -> AddSub11/2
  AddSub8/1 -> Delay4/1
  Delay4/1 -> AddSub5/1
  Constant6/1 -> Mult8/1
  Mult6/1 -> AddSub6/2
  AddSub5/1 -> Delay8/1
  Delay15/1 -> AddSub16/1
  AddSub10/1 -> Delay5/1
  Delay9/1 -> AddSub9/1
  Mult10/1 -> AddSub10/2
  Delay16/1 -> AddSub14/1
  Delay13/1 -> AddSub15/1
  Mult9/1 -> AddSub9/2
  Constant8/1 -> Mult10/1
  Constant15/1 -> Mult15/1
  Constant12/1 -> Mult14/1
  Delay10/1 -> AddSub11/1
  Delay12/1 -> AddSub13/1
  AddSub16/1 -> Delay12/1
  Mult15/1 -> AddSub15/2
  AddSub14/1 -> Delay10/1
  Mult16/1 -> AddSub16/2
  Mult14/1 -> AddSub14/2
  Constant11/1 -> Mult11/1
  Constant9/1 -> Mult9/1
  AddSub15/1 -> Delay15/1
  Constant10/1 -> Mult12/1
  Constant14/1 -> Mult16/1
  In1/1 -> Delay17/1, Mult17/2, Mult15/2, Mult16/2, Mult13/2, Mult14/2, Mult11/2, Mult12/2, Mult9/2, Mult10/2, Mult7/2, Mult8/2, Mult5/2, Mult6/2, Mult3/2, Mult4/2, Mult2/2, Mult1/2
  Delay17/1 -> AddSub17/1
  AddSub17/1 -> Delay13/1
  Mult17/1 -> AddSub17/2
  Constant16/1 -> Mult17/1
  Constant/1 -> Mult2/1
  Delay1/1 -> AddSub1/1
  Mult1/1 -> AddSub1/2
  Constant1/1 -> Mult1/1
  AddSub1/1 -> Delay6/1

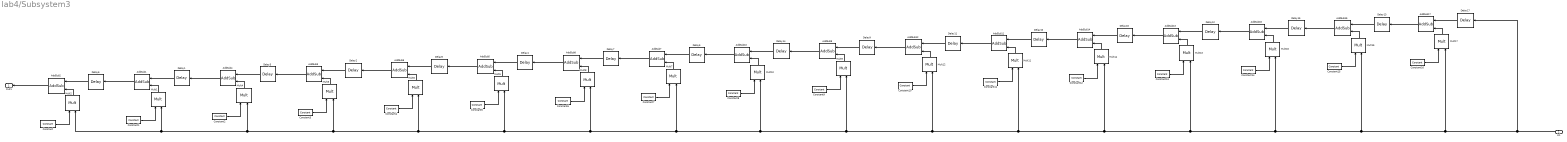
== system lab4/Subsystem3 ==
  In1 : Inport
  AddSub{1..17} (17 alike) : xbsIndex_r4/AddSub  mode=Addition  use_carryin=off  use_carryout=off  en=off  latency=0  precision=User Defined  arith_type="Signed  (2's comp)"  n_bits=17  bin_pt=14  quantization=Truncate  overflow=Wrap  use_behavioral_HDL=off  hw_selection=Fabric  pipelined=off  dbl_ovrd=off  block_type=addsub
  Constant : xbsIndex_r4/Constant  const=h(14,17)  gui_display_data_type=Fixed-point  arith_type=Signed (2's comp)  n_bits=16  bin_pt=14  preci_type=Single  exp_width=8  frac_width=24  explicit_period=off  period=1  equ=P=C  opselect=C  inp2=PCIN>>17  opr=+  inp1=P  carry=CIN  dbl_ovrd=off  block_type=constant
  Constant1 : xbsIndex_r4/Constant  const=h(14,16)  gui_display_data_type=Fixed-point  arith_type=Signed (2's comp)  n_bits=16  bin_pt=14  preci_type=Single  exp_width=8  frac_width=24  explicit_period=off  period=1  equ=P=C  opselect=C  inp2=PCIN>>17  opr=+  inp1=P  carry=CIN  dbl_ovrd=off  block_type=constant
  Constant10 : xbsIndex_r4/Constant  const=h(14,7)  gui_display_data_type=Fixed-point  arith_type=Signed (2's comp)  n_bits=16  bin_pt=14  preci_type=Single  exp_width=8  frac_width=24  explicit_period=off  period=1  equ=P=C  opselect=C  inp2=PCIN>>17  opr=+  inp1=P  carry=CIN  dbl_ovrd=off  block_type=constant
  Constant11 : xbsIndex_r4/Constant  const=h(14,6)  gui_display_data_type=Fixed-point  arith_type=Signed (2's comp)  n_bits=16  bin_pt=14  preci_type=Single  exp_width=8  frac_width=24  explicit_period=off  period=1  equ=P=C  opselect=C  inp2=PCIN>>17  opr=+  inp1=P  carry=CIN  dbl_ovrd=off  block_type=constant
  Constant12 : xbsIndex_r4/Constant  const=h(14,5)  gui_display_data_type=Fixed-point  arith_type=Signed (2's comp)  n_bits=16  bin_pt=14  preci_type=Single  exp_width=8  frac_width=24  explicit_period=off  period=1  equ=P=C  opselect=C  inp2=PCIN>>17  opr=+  inp1=P  carry=CIN  dbl_ovrd=off  block_type=constant
  Constant13 : xbsIndex_r4/Constant  const=h(14,4)  gui_display_data_type=Fixed-point  arith_type=Signed (2's comp)  n_bits=16  bin_pt=14  preci_type=Single  exp_width=8  frac_width=24  explicit_period=off  period=1  equ=P=C  opselect=C  inp2=PCIN>>17  opr=+  inp1=P  carry=CIN  dbl_ovrd=off  block_type=constant
  Constant14 : xbsIndex_r4/Constant  const=h(14,3)  gui_display_data_type=Fixed-point  arith_type=Signed (2's comp)  n_bits=16  bin_pt=14  preci_type=Single  exp_width=8  frac_width=24  explicit_period=off  period=1  equ=P=C  opselect=C  inp2=PCIN>>17  opr=+  inp1=P  carry=CIN  dbl_ovrd=off  block_type=constant
  Constant15 : xbsIndex_r4/Constant  const=h(14,2)  gui_display_data_type=Fixed-point  arith_type=Signed (2's comp)  n_bits=16  bin_pt=14  preci_type=Single  exp_width=8  frac_width=24  explicit_period=off  period=1  equ=P=C  opselect=C  inp2=PCIN>>17  opr=+  inp1=P  carry=CIN  dbl_ovrd=off  block_type=constant
  Constant16 : xbsIndex_r4/Constant  const=h(14,1)  gui_display_data_type=Fixed-point  arith_type=Signed (2's comp)  n_bits=17  bin_pt=14  preci_type=Single  exp_width=8  frac_width=24  explicit_period=off  period=1  equ=P=C  opselect=C  inp2=PCIN>>17  opr=+  inp1=P  carry=CIN  dbl_ovrd=off  block_type=constant
  Constant2 : xbsIndex_r4/Constant  const=h(14,15)  gui_display_data_type=Fixed-point  arith_type=Signed (2's comp)  n_bits=16  bin_pt=14  preci_type=Single  exp_width=8  frac_width=24  explicit_period=off  period=1  equ=P=C  opselect=C  inp2=PCIN>>17  opr=+  inp1=P  carry=CIN  dbl_ovrd=off  block_type=constant
  Constant3 : xbsIndex_r4/Constant  const=h(14,14)  gui_display_data_type=Fixed-point  arith_type=Signed (2's comp)  n_bits=16  bin_pt=14  preci_type=Single  exp_width=8  frac_width=24  explicit_period=off  period=1  equ=P=C  opselect=C  inp2=PCIN>>17  opr=+  inp1=P  carry=CIN  dbl_ovrd=off  block_type=constant
  Constant4 : xbsIndex_r4/Constant  const=h(14,13)  gui_display_data_type=Fixed-point  arith_type=Signed (2's comp)  n_bits=16  bin_pt=14  preci_type=Single  exp_width=8  frac_width=24  explicit_period=off  period=1  equ=P=C  opselect=C  inp2=PCIN>>17  opr=+  inp1=P  carry=CIN  dbl_ovrd=off  block_type=constant
  Constant5 : xbsIndex_r4/Constant  const=h(14,12)  gui_display_data_type=Fixed-point  arith_type=Signed (2's comp)  n_bits=16  bin_pt=14  preci_type=Single  exp_width=8  frac_width=24  explicit_period=off  period=1  equ=P=C  opselect=C  inp2=PCIN>>17  opr=+  inp1=P  carry=CIN  dbl_ovrd=off  block_type=constant
  Constant6 : xbsIndex_r4/Constant  const=h(14,11)  gui_display_data_type=Fixed-point  arith_type=Signed (2's comp)  n_bits=16  bin_pt=14  preci_type=Single  exp_width=8  frac_width=24  explicit_period=off  period=1  equ=P=C  opselect=C  inp2=PCIN>>17  opr=+  inp1=P  carry=CIN  dbl_ovrd=off  block_type=constant
  Constant7 : xbsIndex_r4/Constant  const=h(14,10)  gui_display_data_type=Fixed-point  arith_type=Signed (2's comp)  n_bits=16  bin_pt=14  preci_type=Single  exp_width=8  frac_width=24  explicit_period=off  period=1  equ=P=C  opselect=C  inp2=PCIN>>17  opr=+  inp1=P  carry=CIN  dbl_ovrd=off  block_type=constant
  Constant8 : xbsIndex_r4/Constant  const=h(14,9)  gui_display_data_type=Fixed-point  arith_type=Signed (2's comp)  n_bits=16  bin_pt=14  preci_type=Single  exp_width=8  frac_width=24  explicit_period=off  period=1  equ=P=C  opselect=C  inp2=PCIN>>17  opr=+  inp1=P  carry=CIN  dbl_ovrd=off  block_type=constant
  Constant9 : xbsIndex_r4/Constant  const=h(14,8)  gui_display_data_type=Fixed-point  arith_type=Signed (2's comp)  n_bits=16  bin_pt=14  preci_type=Single  exp_width=8  frac_width=24  explicit_period=off  period=1  equ=P=C  opselect=C  inp2=PCIN>>17  opr=+  inp1=P  carry=CIN  dbl_ovrd=off  block_type=constant
  Delay{1..17} (17 alike) : xbsIndex_r4/Delay  rst=off  infoeditControl=Selection of Reset will increase slice count due to use of real FFs and instead of SRLs  en=off  latency=1  reg_retiming=off  dbl_ovrd=off  block_type=delay
  Mult{1..17} (17 alike) : xbsIndex_r4/Mult  precision=User Defined  arith_type="Signed  (2's comp)"  n_bits=16  bin_pt=14  quantization="Round  (unbiased: +/- Inf)"  overflow=Flag as error  en=off  latency=0  use_behavioral_HDL=off  opt=Speed  use_embedded=on  optimum_pipeline=off  pipeline=on  dbl_ovrd=off  use_rpm=on  placement_style=Triangular  block_type=mult
  Out1 : Outport
  wires:
  Mult2/1 -> AddSub2/2
  AddSub2/1 -> Out1/1
  Delay6/1 -> AddSub2/1
  Constant2/1 -> Mult4/1
  AddSub4/1 -> Delay1/1
  Mult4/1 -> AddSub4/2
  Delay3/1 -> AddSub4/1
  Constant4/1 -> Mult6/1
  AddSub12/1 -> Delay9/1
  Constant3/1 -> Mult3/1
  Mult13/1 -> AddSub13/2
  AddSub13/1 -> Delay16/1
  Delay7/1 -> AddSub8/1
  Constant13/1 -> Mult13/1
  Mult3/1 -> AddSub3/2
  Mult8/1 -> AddSub8/2
  Delay8/1 -> AddSub6/1
  Delay2/1 -> AddSub3/1
  AddSub3/1 -> Delay3/1
  Delay14/1 -> AddSub10/1
  AddSub11/1 -> Delay11/1
  AddSub9/1 -> Delay14/1
  AddSub6/1 -> Delay2/1
  Delay5/1 -> AddSub7/1
  Constant7/1 -> Mult7/1
  Mult5/1 -> AddSub5/2
  Constant5/1 -> Mult5/1
  Mult12/1 -> AddSub12/2
  Mult7/1 -> AddSub7/2
  AddSub7/1 -> Delay7/1
  Delay11/1 -> AddSub12/1
  Mult11/1 -> AddSub11/2
  AddSub8/1 -> Delay4/1
  Delay4/1 -> AddSub5/1
  Constant6/1 -> Mult8/1
  Mult6/1 -> AddSub6/2
  AddSub5/1 -> Delay8/1
  Delay15/1 -> AddSub16/1
  AddSub10/1 -> Delay5/1
  Delay9/1 -> AddSub9/1
  Mult10/1 -> AddSub10/2
  Delay16/1 -> AddSub14/1
  Delay13/1 -> AddSub15/1
  Mult9/1 -> AddSub9/2
  Constant8/1 -> Mult10/1
  Constant15/1 -> Mult15/1
  Constant12/1 -> Mult14/1
  Delay10/1 -> AddSub11/1
  Delay12/1 -> AddSub13/1
  AddSub16/1 -> Delay12/1
  Mult15/1 -> AddSub15/2
  AddSub14/1 -> Delay10/1
  Mult16/1 -> AddSub16/2
  Mult14/1 -> AddSub14/2
  Constant11/1 -> Mult11/1
  Constant9/1 -> Mult9/1
  AddSub15/1 -> Delay15/1
  Constant10/1 -> Mult12/1
  Constant14/1 -> Mult16/1
  In1/1 -> Delay17/1, Mult17/2, Mult15/2, Mult16/2, Mult13/2, Mult14/2, Mult11/2, Mult12/2, Mult9/2, Mult10/2, Mult7/2, Mult8/2, Mult5/2, Mult6/2, Mult3/2, Mult4/2, Mult2/2, Mult1/2
  Delay17/1 -> AddSub17/1
  AddSub17/1 -> Delay13/1
  Mult17/1 -> AddSub17/2
  Constant16/1 -> Mult17/1
  Constant/1 -> Mult2/1
  Delay1/1 -> AddSub1/1
  Mult1/1 -> AddSub1/2
  Constant1/1 -> Mult1/1
  AddSub1/1 -> Delay6/1
